simulink model "ar2_orient_456"  (R2019b)
settings: Solver=VariableStepAuto  StartTime=0.0  StopTime=10.0  RelTol=1e-3
libraries: simulink_extras x9
settings Model: Creator=ah501846  LastModifiedBy=ah501846

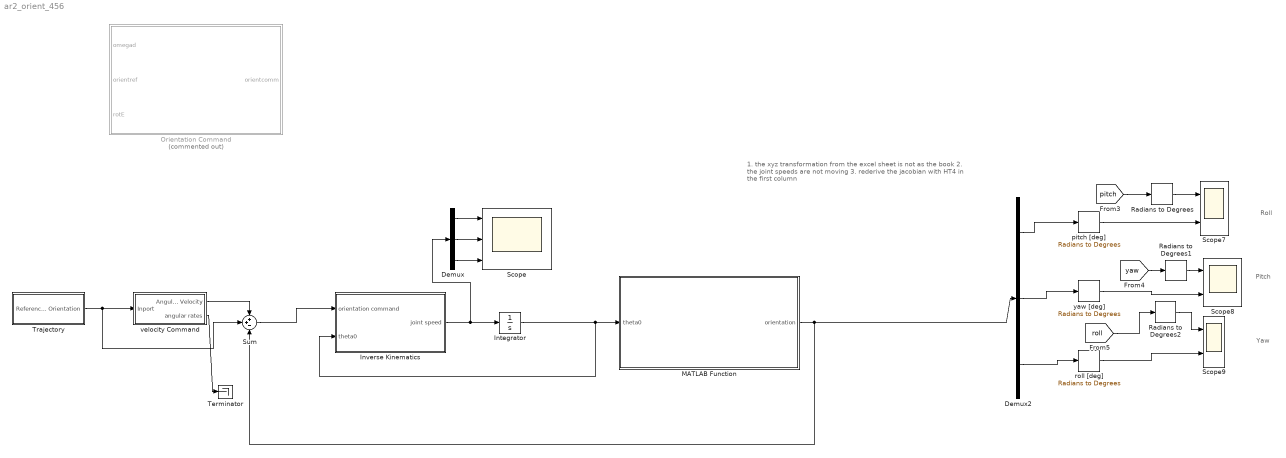
== system ar2_orient_456 ==
  note: 1. the xyz transformation from the excel sheet is not as the book
      | 2. the joint speeds are not moving
      | 3. rederive the jacobian with HT4 in the first column
  note: Pitch
  note: Roll
  note: Yaw
  Demux : Demux  Outputs=3
  Demux2 : Demux  Outputs=3
  Integrator : Integrator  InitialCondition=[20 20 20]*pi/180
  Inverse Kinematics : Subsystem
  MATLAB Function : MATLAB Function  TreatAsAtomicUnit=on
  Orientation Command : MATLAB Function  Commented=on  TreatAsAtomicUnit=on
  Radians to Degrees : simulink_extras/Transformations/Radians to Degrees
  Radians to Degrees1 : simulink_extras/Transformations/Radians to Degrees
  Radians to Degrees2 : simulink_extras/Transformations/Radians to Degrees
  Scope : Scope  NumInputPorts=3
  Scope7 : Scope  NumInputPorts=2
  Scope8 : Scope  NumInputPorts=2
  Scope9 : Scope  NumInputPorts=2
  Sum : Sum  Inputs=++-
  Terminator : Terminator
  "Trajectory " : Subsystem
  pitch [deg] : simulink_extras/Transformations/Radians to Degrees
  roll [deg] : simulink_extras/Transformations/Radians to Degrees
  velocity Command : Subsystem
  yaw [deg] : simulink_extras/Transformations/Radians to Degrees
  wires:
  Inverse Kinematics/1(joint speed) -> Demux/1, Integrator/1
  pitch [deg]/1 -> Scope7/2
  Demux2/2 -> yaw [deg]/1
  [yaw] -> Radians to Degrees1/1
  Radians to Degrees1/1 -> Scope8/1
  Radians to Degrees/1 -> Scope7/1
  MATLAB Function/1(orientation) -> Demux2/1, Sum/3
  [pitch] -> Radians to Degrees/1
  Radians to Degrees2/1 -> Scope9/1
  [roll] -> Radians to Degrees2/1
  roll [deg]/1 -> Scope9/2
  yaw [deg]/1 -> Scope8/2
  Demux2/1 -> pitch [deg]/1
  Demux2/3 -> roll [deg]/1
  Integrator/1 -> Inverse Kinematics/2(theta0), MATLAB Function/1(theta0)
  ? -> Orientation Command/1(omegad)
  ? -> Orientation Command/2(orientref)
  Demux/1 -> Scope/1
  Demux/2 -> Scope/2
  Demux/3 -> Scope/3
  "Trajectory "/1(Reference Orientation) -> Sum/2, velocity Command/1(Inport)
  velocity Command/1(Angular Velocity) -> Sum/1
  velocity Command/2(angular rates) -> Terminator/1
  Sum/1 -> Inverse Kinematics/1(orientation command)

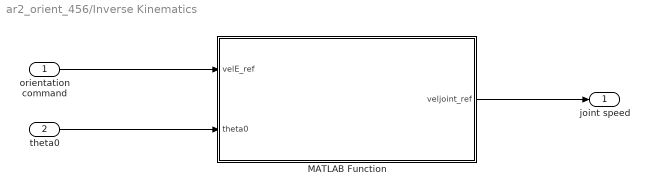
== system ar2_orient_456/Inverse Kinematics ==
  orientation command : Inport
  theta0 : Inport  Port=2
  MATLAB Function : MATLAB Function  TreatAsAtomicUnit=on
  joint speed : Outport  VectorParamsAs1DForOutWhenUnconnected=off
  wires:
  MATLAB Function/1(veljoint_ref) -> joint speed/1
  theta0/1 -> MATLAB Function/2(theta0)
  orientation command/1 -> MATLAB Function/1(velE_ref)

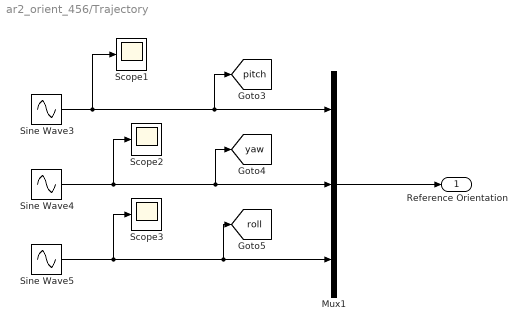
== system ar2_orient_456/Trajectory  ==
  Mux1 : Mux  Inputs=3
  Scope1 : Scope
  Scope2 : Scope
  Scope3 : Scope
  Sine Wave3 : Sin  Amplitude=5*pi/180  Bias=20*pi/180  Frequency=2*pi/100/4  SampleTime=0
  Sine Wave4 : Sin  Amplitude=5*pi/180  Bias=20*pi/180  Frequency=2*pi/100/4  SampleTime=0
  Sine Wave5 : Sin  Amplitude=5*pi/180  Bias=20*pi/180  Frequency=2*pi/100/4  SampleTime=0
  Reference Orientation : Outport
  tag scope: pitch=global, roll=global, yaw=global
  wires:
  Sine Wave5/1 -> Scope3/1, [roll], Mux1/3
  Sine Wave4/1 -> Scope2/1, [yaw], Mux1/2
  Sine Wave3/1 -> Scope1/1, [pitch], Mux1/1
  Mux1/1 -> Reference Orientation/1

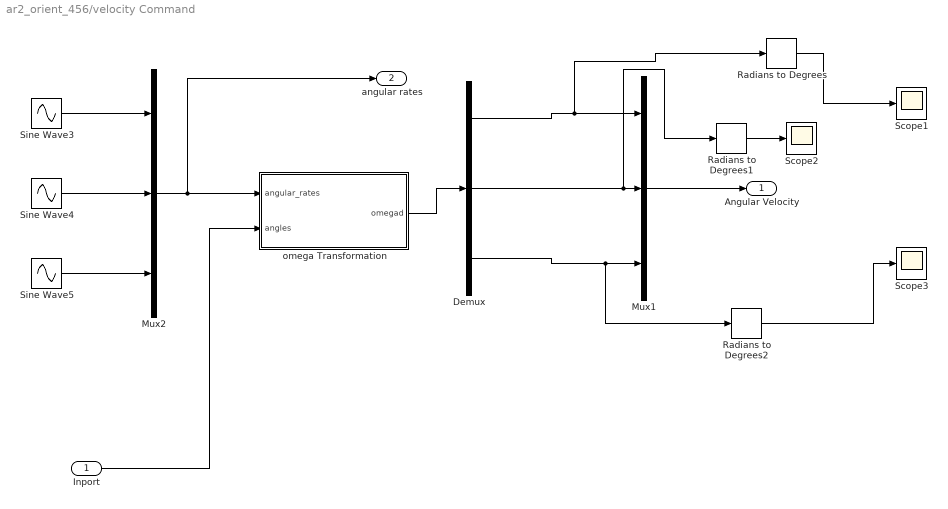
== system ar2_orient_456/velocity Command ==
  Inport : Inport
  Demux : Demux  Outputs=3
  Mux1 : Mux  Inputs=3
  Mux2 : Mux  Inputs=3
  Radians to Degrees : simulink_extras/Transformations/Radians to Degrees
  Radians to Degrees1 : simulink_extras/Transformations/Radians to Degrees
  Radians to Degrees2 : simulink_extras/Transformations/Radians to Degrees
  Scope1 : Scope
  Scope2 : Scope
  Scope3 : Scope
  Sine Wave3 : Sin  Amplitude=5*pi/180  Frequency=2*pi/100/4  Phase=pi/2  SampleTime=0
  Sine Wave4 : Sin  Amplitude=5*pi/180  Frequency=2*pi/100/4  Phase=pi/2  SampleTime=0
  Sine Wave5 : Sin  Amplitude=5*pi/180  Frequency=2*pi/100/4  Phase=pi/2  SampleTime=0
  omega Transformation : MATLAB Function  TreatAsAtomicUnit=on
  Angular Velocity : Outport
  angular rates : Outport  Port=2
  wires:
  Mux1/1 -> Angular Velocity/1
  Mux2/1 -> angular rates/1, omega Transformation/1(angular_rates)
  Demux/2 -> Radians to Degrees1/1, Mux1/2
  Demux/1 -> Radians to Degrees/1, Mux1/1
  Demux/3 -> Radians to Degrees2/1, Mux1/3
  Sine Wave3/1 -> Mux2/1
  Sine Wave5/1 -> Mux2/3
  Sine Wave4/1 -> Mux2/2
  Radians to Degrees/1 -> Scope1/1
  Radians to Degrees1/1 -> Scope2/1
  Radians to Degrees2/1 -> Scope3/1
  omega Transformation/1(omegad) -> Demux/1
  Inport/1 -> omega Transformation/2(angles)

== matlab function ar2_orient_456/MATLAB Function ==
  data: orientation output; theta0 input
% function to calculate analytical Jacobian
function orientation  = manipFK(theta0)
%% Inputs
theta4 = theta0(1);
theta5 = theta0(2);
theta6 = theta0(3);
cth4 = cos(theta4);
cth5 = cos(theta5);
cth6 = cos(theta6);
sth4 = sin(theta4);
sth5 = sin(theta5);
sth6 = sin(theta6);
%% Direct Forward Kinematics
HT3 = [cth4*cth5*cth6 - sth4*sth6   -cth6*sth4 - cth4*cth5*sth6     cth4*sth5  ;
    cth4*sth6 + cth5*cth6*sth4   cth4*cth6 - cth5*sth4*sth6      sth4*sth5   ;
    -cth6*sth5                       sth5*sth6                   cth5     ];


nu = atan2(sqrt(HT3(1,3)^2+HT3(2,3)^2), HT3(3,3));
psi = atan2(HT3(3,2),-HT3(3,1));
phi = atan2(HT3(2,3),HT3(1,3));
%% Outputs
orientation = [phi nu psi]';

== matlab function ar2_orient_456/Inverse Kinematics/MATLAB Function ==
  data: velE_ref input; veljoint_ref output; theta0 input
function veljoint_ref = trajectoryIK(velE_ref,theta0)
theta4 = theta0(1);
theta5 = theta0(2);
cth4 = cos(theta4);
cth5 = cos(theta5);
sth4 = sin(theta4);
sth5 = sin(theta5);

J_rot = [0  -sth4   cth4*sth5;
         0  cth4    sth4*sth5;
         1   0      cth5];
     
     



veljoint_ref = pinv(J_rot) * velE_ref;

== matlab function ar2_orient_456/Orientation Command ==
  data: omegad input; orientref input; rotE input; orientcomm output
function orientcomm = orientCommand(omegad, orientref, rotE)

phi = orientref(1);
nu = orientref(2);
psi = orientref(3);
%ZYZ rotation
% rotD = [cos(phi)*cos(nu)*cos(psi)-sin(phi)*sin(psi)    -cos(phi)*cos(nu)*sin(psi)-sin(phi)*cos(psi)   cos(phi)*sin(nu);
%     sin(phi)*cos(nu)*cos(psi)+cos(phi)*sin(psi)    -sin(phi)*cos(nu)*sin(psi)+cos(phi)*cos(psi)   sin(phi)*sin(nu);
%     -sin(nu)*cos(psi)    sin(nu)*sin(psi)  cos(nu)];

%XYZ rotation
rotD = [cos(phi)*cos(nu)    cos(phi)*sin(nu)*sin(psi)-sin(phi)*cos(psi)     cos(phi)*sin(nu)*cos(psi)+sin(phi)*sin(psi);
        sin(phi)*cos(nu)    sin(phi)*sin(nu)*sin(psi)+cos(phi)*cos(psi)     sin(phi)*sin(nu)*cos(psi)-cos(phi)*sin(psi);
        -sin(nu)            cos(nu)*sin(psi)                                cos(nu)*cos(psi)];

nd = rotD(1:3,1);
sd = rotD(1:3,2);
ad = rotD(1:3,3);

ne = rotE(1:3,1);
se = rotE(1:3,2);
ae = rotE(1:3,3);


% nu_f = acos(trace(Rif)-1)/2;
% r = 0.5/sin(nu) * [Rif(3,2) - Rif(2,3);
%                    Rif(1,3) - Rif(3,1); 
%                    Rif(2,1) - Rif(1,2)];  %sin nu neq 0

% nu_f = deg2rad(0.9181);
% r = [-0.2654 -0.2780 1.1910]';
% 
% rx = r(1);
% ry = r(2);
% rz = r(3);




S_nd = [0       -nd(3)      nd(2);
    nd(3)       0       -nd(1);
    -nd(2)      nd(1)       0];
S_sd = [0       -sd(3)      sd(2);
    sd(3)       0       -sd(1);
    -sd(2)      sd(1)       0];
S_ad = [0       -ad(3)      ad(2);
    ad(3)       0       -ad(1);
    -ad(2)      ad(1)       0];
S_ne = [0       -ne(3)      ne(2);
    ne(3)       0       -ne(1);
    -ne(2)      ne(1)       0];
S_se = [0       -se(3)      se(2);
    se(3)       0       -se(1);
    -se(2)      se(1)       0];
S_ae = [0       -ae(3)      ae(2);
    ae(3)       0       -ae(1);
    -ae(2)      ae(1)       0];



% if ne'*nd < 0 || se'*sd < 0 || ae'*ad < 0
%     disp("ne'*nd is not geq 0");
% else
%     eo = 0.5*(cross(ne,nd) + cross(se,sd) + cross(ae,ad));
% end

eo = 0.5*(cross(ne,nd) + cross(se,sd) + cross(ae,ad));
% eo = ne.*nd + se.*sd + ae.*ad;
L = -0.5*(S_nd*S_ne + S_sd*S_se + S_ad*S_ae);
Ko = [10  0  0;
    0  10  0;
    0  0  10];
orientcomm = pinv(L)*(L' * omegad + Ko*eo);
% orientcomm = eo;
% orientcomm = omegad;

% orientcomm = omegad + Ko*eo;

== matlab function ar2_orient_456/velocity Command/omega Transformation ==
  data: angular_rates input; omegad output; angles input
% ZYZ notation used here
% Disambiguation: psi is also used for the GV heading

function omegad = omegaTrans(angular_rates, angles)
phi = angles(1);
nu = angles(2);
psi = angles(3);

% nu = atan2(sqrt(HT3(1,3)^2+HT3(2,3)^2), HT3(3,3)); %theta5
% phi = atan2(HT3(2,3), HT3(1,3));    %theta4
% psi = atan2(HT3(3,2), -HT3(3,1));   %theta6

% %ZYZ
% T = [0 -sin(phi) cos(phi)*sin(nu);
%      0  cos(phi) sin(phi)*sin(nu);
%      1  0   cos(nu)];

%XYZ
% T = [cos(phi)*cos(psi) sin(psi) 0;
%      -cos(phi)*sin(psi) cos(psi) 0;
%      sin(psi) 0 1];

T = [0     -sth4   cth4*sth5;
      0     cth4    sth4*sth5;
      1      0          cth5];
 
omegad = T * angular_rates;
% omegad = [0 0 0]';
